simulink model "Utkarsh_2005574_W1_P3"  (R2020b)
settings: Solver=FixedStepDiscrete  StartTime=0.0  StopTime=10.0  RelTol=1e-3
settings Model: Creator=home  LastModifiedBy=home

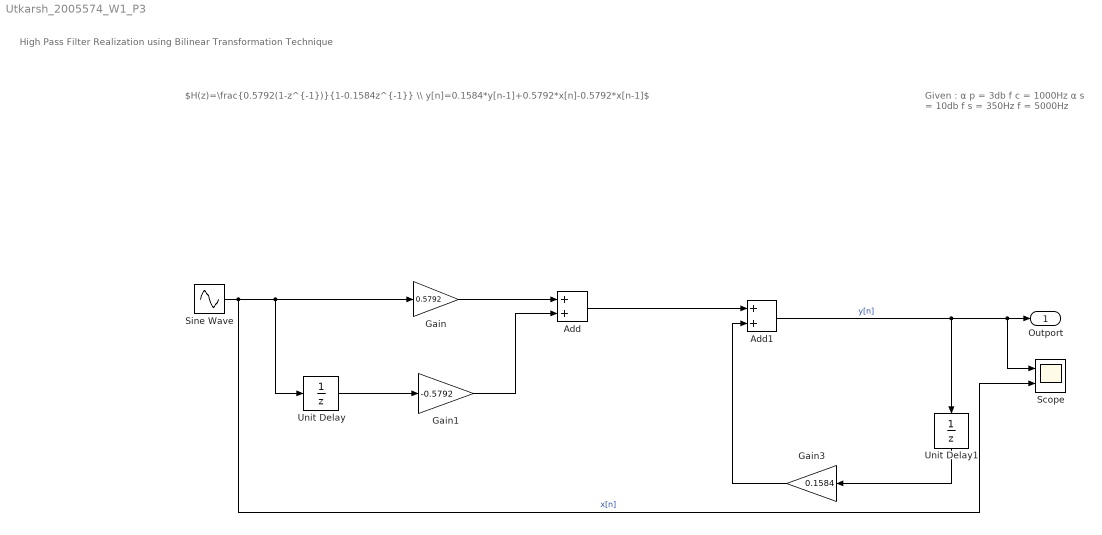
== system Utkarsh_2005574_W1_P3 ==
  note: $H(z)=\frac{0.5792(1-z^{-1})}{1-0.1584z^{-1}} \\ y[n]=0.1584*y[n-1]+0.5792*x[n]-0.5792*x[n-1]$
  note: Given :
      | α p = 3db
      | f c = 1000Hz
      | α s = 10db
      | f s = 350Hz
      | f = 5000Hz
  note: High Pass Filter Realization using Bilinear Transformation Technique
  Add : Sum
  Add1 : Sum
  Gain : Gain  Gain=0.5792
  Gain1 : Gain  Gain=-0.5792
  Gain3 : Gain  Gain=0.1584
  Scope : Scope  NumInputPorts=2
  Sine Wave : Sin  Amplitude=2  Frequency=2*pi*10000  SampleTime=0
  Unit Delay : UnitDelay  SampleTime=-1  HasFrameUpgradeWarning=on
  Unit Delay1 : UnitDelay  SampleTime=-1  HasFrameUpgradeWarning=on
  Outport : Outport
  wires:
  Gain/1 -> Add/1
  Sine Wave/1 -> Scope/2, Unit Delay/1, Gain/1  "x[n]"
  Unit Delay/1 -> Gain1/1
  Gain1/1 -> Add/2
  Unit Delay1/1 -> Gain3/1
  Add/1 -> Add1/1
  Gain3/1 -> Add1/2
  Add1/1 -> Scope/1, Outport/1, Unit Delay1/1  "y[n]"
